simulink model "robust_drift_REALTIME"  (R2020b)
settings: Solver=VariableStepAuto  StartTime=0.0  StopTime=10.0  RelTol=1e-3
values from neighbouring files (symbols this model uses):
  drv =     [balrob_params.mat]
  gbox =     [balrob_params.mat]    (also in sfun_balrob_long_dyn.m = block.DialogPrm(4).Data)
  sens =     [balrob_params.mat]
  Ts = 0.01    [balrob_params.mat]
  wheel =     [balrob_params.mat]    (also in sfun_balrob_long_dyn.m = block.DialogPrm(5).Data)
undefined symbols (not defined in the file or in its folder): C_gain, denHw, denLPFz, DiscIntNeverNeededParam, Ki, N_u, N_x, numHw, numLPFz, T
settings Model: Creator=39345  LastModifiedBy=39345

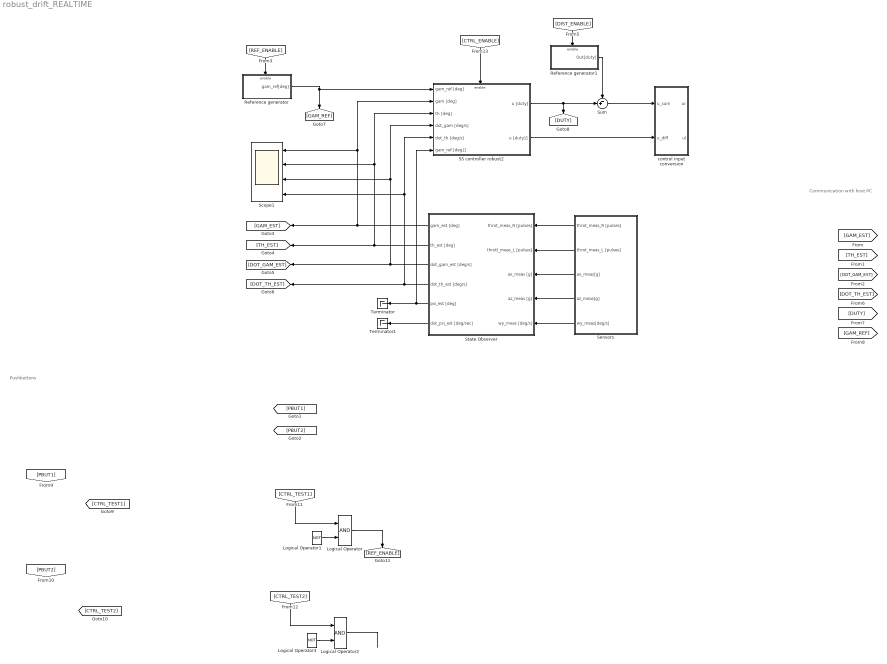
== system robust_drift_REALTIME ==
  note: Communication with host PC
  note: Pushbuttons
  Logical Operator : Logic  AllPortsSameDT=off  OutDataTypeStr=boolean
  Logical Operator1 : Logic  Operator=NOT  Inputs=1  AllPortsSameDT=off  OutDataTypeStr=boolean
  Logical Operator2 : Logic  AllPortsSameDT=off  OutDataTypeStr=boolean
  Logical Operator3 : Logic  Operator=NOT  Inputs=1  AllPortsSameDT=off  OutDataTypeStr=boolean
  Reference generator : Subsystem
  Reference generator1 : Subsystem
  SS controller robust2 : Subsystem
  Scope1 : Scope  NumInputPorts=4
  Sensors : Subsystem
  State Observer : Subsystem
  Sum : Sum  Inputs=-+|
  Terminator : Terminator
  Terminator1 : Terminator
  control input conversion : Subsystem
  wires:
  Logical Operator/1 -> [REF_ENABLE]
  [CTRL_TEST1] -> Logical Operator/1
  Logical Operator2/1 -> ?
  Logical Operator1/1 -> Logical Operator/2
  [CTRL_TEST2] -> Logical Operator2/1
  Logical Operator3/1 -> Logical Operator2/2
  [CTRL_ENABLE] -> SS controller robust2/Enable
  State Observer/5(psi_est [deg]) -> SS controller robust2/6(gam_ref [deg]1), Terminator/1
  [REF_ENABLE] -> Reference generator/Enable
  State Observer/1(gam_est [deg]) -> SS controller robust2/2(gam [deg]), Scope1/1, [GAM_EST]
  Sensors/3(ax_meas[g]) -> State Observer/3("ax_meas [g] ")
  State Observer/2(th_est [deg]) -> SS controller robust2/3(th [deg]), Scope1/2, [TH_EST]
  Sensors/4(az_meas[g]) -> State Observer/4("az_meas [g] ")
  Reference generator/1(gam_ref[deg]) -> SS controller robust2/1(gam_ref [deg]), [GAM_REF]
  Sum/1 -> control input conversion/1(u_sum)
  Sensors/2(throt_meas_L [pulses]) -> State Observer/2(throtl_meas_L [pulses])
  State Observer/4(dot_th_est [deg/s]) -> SS controller robust2/5(dot_th [deg/s]), Scope1/4, [DOT_TH_EST]
  Reference generator1/1(Out[duty]) -> Sum/1
  State Observer/6(dot_psi_est [deg/sec]) -> Terminator1/1
  Sensors/1(throt_meas_R [pulses]) -> State Observer/1("throt_meas_R [pulses] ")
  State Observer/3(dot_gam_est [deg/s]) -> SS controller robust2/4(dot_gam [deg/s]), Scope1/3, [DOT_GAM_EST]
  Sensors/5(wy_meas[deg/s]) -> State Observer/5(wy_meas [deg/s])
  [DIST_ENABLE] -> Reference generator1/Enable
  SS controller robust2/1(u [duty]) -> Sum/2, [DUTY]
  SS controller robust2/2(u [duty]1) -> control input conversion/2(u_diff)

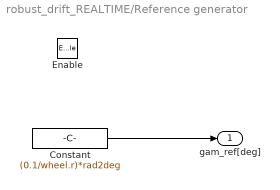
== system robust_drift_REALTIME/Reference generator ==
  Enable : EnablePort  StatesWhenEnabling=reset
  Constant : Constant  Value=(0.1/wheel.r)*rad2deg
  gam_ref[deg] : Outport
  wires:
  Constant/1 -> gam_ref[deg]/1

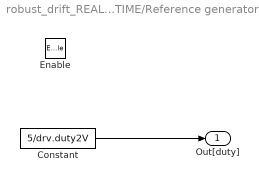
== system robust_drift_REALTIME/Reference generator1 ==
  Enable : EnablePort  StatesWhenEnabling=reset
  Constant : Constant  Value=5/drv.duty2V
  Out[duty] : Outport
  wires:
  Constant/1 -> Out[duty]/1

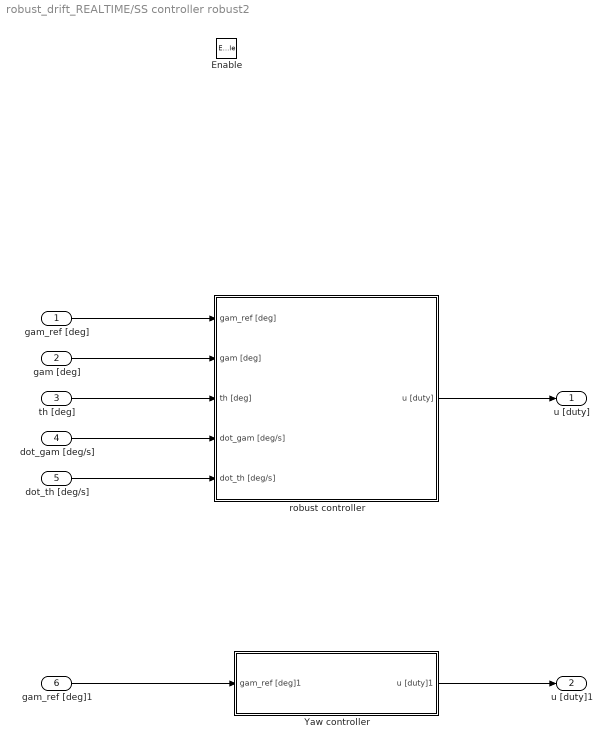
== system robust_drift_REALTIME/SS controller robust2 ==
  gam_ref [deg] : Inport
  gam [deg] : Inport  Port=2
  th [deg] : Inport  Port=3
  dot_gam [deg/s] : Inport  Port=4
  dot_th [deg/s] : Inport  Port=5
  gam_ref [deg]1 : Inport  Port=6
  Enable : EnablePort
  Yaw controller : Subsystem
  robust controller : Subsystem
  u [duty] : Outport
  u [duty]1 : Outport  Port=2
  wires:
  gam_ref [deg]1/1 -> Yaw controller/1(gam_ref [deg]1)
  Yaw controller/1(u [duty]1) -> u [duty]1/1
  gam_ref [deg]/1 -> robust controller/1(gam_ref [deg])
  robust controller/1(u [duty]) -> u [duty]/1
  gam [deg]/1 -> robust controller/2(gam [deg])
  th [deg]/1 -> robust controller/3(th [deg])
  dot_gam [deg/s]/1 -> robust controller/4(dot_gam [deg/s])
  dot_th [deg/s]/1 -> robust controller/5(dot_th [deg/s])

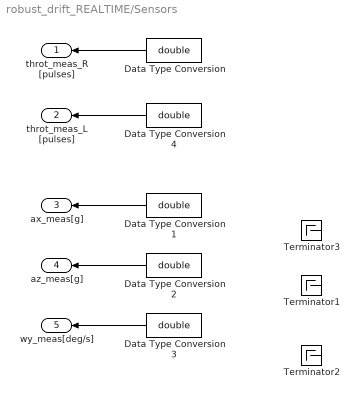
== system robust_drift_REALTIME/Sensors ==
  Data Type Conversion{,1..4} (5 alike) : DataTypeConversion  OutDataTypeStr=double
  Terminator1 : Terminator
  Terminator2 : Terminator
  Terminator3 : Terminator
  throt_meas_R [pulses] : Outport
  throt_meas_L [pulses] : Outport  Port=2
  ax_meas[g] : Outport  Port=3
  az_meas[g] : Outport  Port=4
  wy_meas[deg/s] : Outport  Port=5
  wires:
  Data Type Conversion/1 -> throt_meas_R [pulses]/1
  Data Type Conversion1/1 -> ax_meas[g]/1
  Data Type Conversion2/1 -> az_meas[g]/1
  Data Type Conversion3/1 -> wy_meas[deg/s]/1
  Data Type Conversion4/1 -> throt_meas_L [pulses]/1

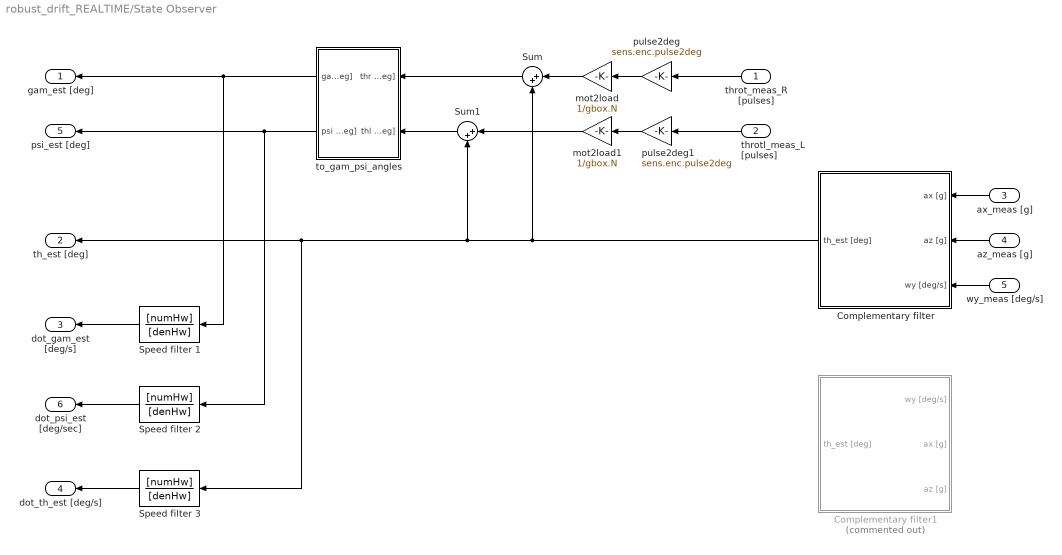
== system robust_drift_REALTIME/State Observer ==
  "throt_meas_R [pulses] " : Inport
  throtl_meas_L [pulses] : Inport  Port=2
  "ax_meas [g] " : Inport  Port=3
  "az_meas [g] " : Inport  Port=4
  wy_meas [deg/s] : Inport  Port=5
  Complementary filter : Subsystem
  Complementary filter1 : Subsystem  Commented=on
  Speed filter 1 : DiscreteTransferFcn  Numerator=[numHw]  Denominator=[denHw]  SampleTime=Ts
  Speed filter 2 : DiscreteTransferFcn  Numerator=[numHw]  Denominator=[denHw]  SampleTime=Ts
  Speed filter 3 : DiscreteTransferFcn  Numerator=[numHw]  Denominator=[denHw]  SampleTime=Ts
  Sum : Sum  Inputs=|++
  Sum1 : Sum  Inputs=|++
  mot2load : Gain  Gain=1/gbox.N
  mot2load1 : Gain  Gain=1/gbox.N
  pulse2deg : Gain  Gain=sens.enc.pulse2deg
  pulse2deg1 : Gain  Gain=sens.enc.pulse2deg
  to_gam_psi_angles : Subsystem
  gam_est [deg] : Outport
  th_est [deg] : Outport  Port=2
  dot_gam_est [deg/s] : Outport  Port=3
  dot_th_est [deg/s] : Outport  Port=4
  psi_est [deg] : Outport  Port=5
  dot_psi_est [deg/sec] : Outport  Port=6
  wires:
  pulse2deg/1 -> mot2load/1
  "throt_meas_R [pulses] "/1 -> pulse2deg/1
  mot2load/1 -> Sum/1
  Complementary filter/1("th_est [deg] ") -> Sum/2, th_est [deg]/1, Speed filter 3/1, Sum1/2
  Speed filter 1/1 -> dot_gam_est [deg/s]/1
  Speed filter 3/1 -> dot_th_est [deg/s]/1
  "ax_meas [g] "/1 -> Complementary filter/1("ax [g] ")
  "az_meas [g] "/1 -> Complementary filter/2("az [g] ")
  wy_meas [deg/s]/1 -> Complementary filter/3(wy [deg/s])
  throtl_meas_L [pulses]/1 -> pulse2deg1/1
  pulse2deg1/1 -> mot2load1/1
  mot2load1/1 -> Sum1/1
  Sum1/1 -> to_gam_psi_angles/2(thl [deg])
  Sum/1 -> to_gam_psi_angles/1(thr [deg])
  to_gam_psi_angles/1(gam [deg]) -> Speed filter 1/1, gam_est [deg]/1
  to_gam_psi_angles/2(psi [deg]) -> Speed filter 2/1, psi_est [deg]/1
  Speed filter 2/1 -> dot_psi_est [deg/sec]/1

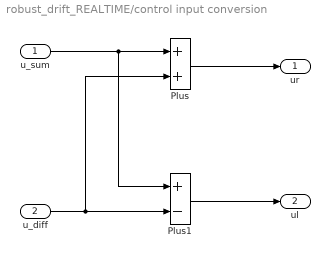
== system robust_drift_REALTIME/control input conversion ==
  u_sum : Inport
  u_diff : Inport  Port=2
  Plus : Sum
  Plus1 : Sum  Inputs=+-
  ur : Outport
  ul : Outport  Port=2
  wires:
  u_sum/1 -> Plus1/1, Plus/1
  u_diff/1 -> Plus1/2, Plus/2
  Plus/1 -> ur/1
  Plus1/1 -> ul/1

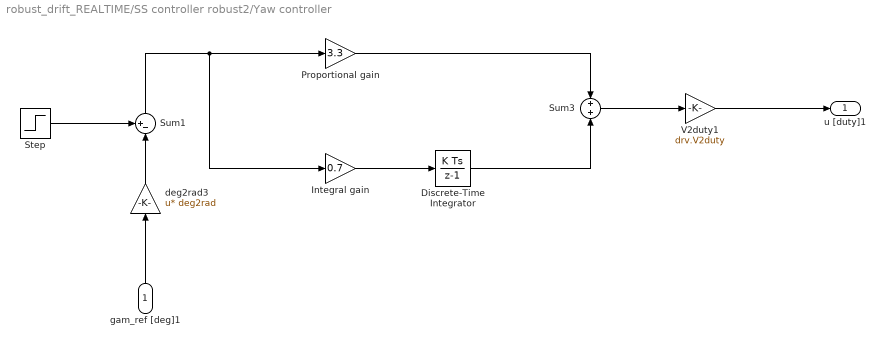
== system robust_drift_REALTIME/SS controller robust2/Yaw controller ==
  gam_ref [deg]1 : Inport
  Discrete-Time Integrator : DiscreteIntegrator  SampleTime=-1  ICPrevOutput=DiscIntNeverNeededParam  ICPrevScaledInput=DiscIntNeverNeededParam
  Integral gain : Gain  Gain=0.7
  Proportional gain : Gain  Gain=3.3
  Step : Step  Time=0  After=0  SampleTime=0
  Sum1 : Sum  Inputs=+-|
  Sum3 : Sum  Inputs=+|+
  V2duty1 : Gain  Gain=drv.V2duty
  deg2rad3 : Gain  Gain=deg2rad  Multiplication=Matrix(u*K)
  u [duty]1 : Outport
  wires:
  gam_ref [deg]1/1 -> deg2rad3/1
  Sum1/1 -> Integral gain/1, Proportional gain/1
  Step/1 -> Sum1/1
  Integral gain/1 -> Discrete-Time Integrator/1
  deg2rad3/1 -> Sum1/2
  V2duty1/1 -> u [duty]1/1
  Proportional gain/1 -> Sum3/1
  Discrete-Time Integrator/1 -> Sum3/2
  Sum3/1 -> V2duty1/1

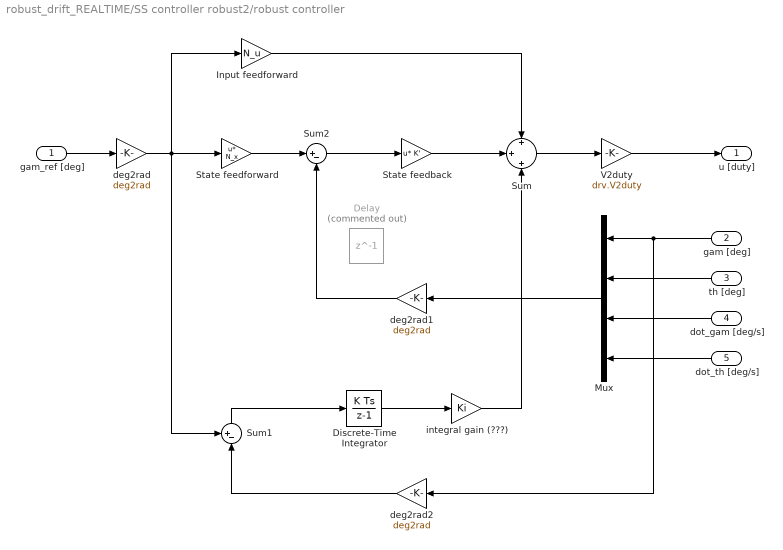
== system robust_drift_REALTIME/SS controller robust2/robust controller ==
  gam_ref [deg] : Inport
  gam [deg] : Inport  Port=2
  th [deg] : Inport  Port=3
  dot_gam [deg/s] : Inport  Port=4
  dot_th [deg/s] : Inport  Port=5
  Delay : Delay  Commented=on  DelayLength=1  InitialCondition=0
  Discrete-Time Integrator : DiscreteIntegrator  SampleTime=0.01  ICPrevOutput=DiscIntNeverNeededParam  ICPrevScaledInput=DiscIntNeverNeededParam
  Input feedforward : Gain  Gain=N_u
  Mux : Mux
  State feedback : Gain  Gain=K'  Multiplication=Matrix(u*K)
  "State feedforward\t" : Gain  Gain=N_x  Multiplication=Matrix(u*K)
  Sum : Sum  Inputs=+|+|+
  Sum1 : Sum  Inputs=+-|
  Sum2 : Sum  Inputs=|+-
  V2duty : Gain  Gain=drv.V2duty
  deg2rad : Gain  Gain=deg2rad
  deg2rad1 : Gain  Gain=deg2rad
  deg2rad2 : Gain  Gain=deg2rad
  integral gain (???) : Gain  Gain=Ki
  u [duty] : Outport
  wires:
  integral gain (???)/1 -> Sum/3
  deg2rad2/1 -> Sum1/2
  Sum1/1 -> Discrete-Time Integrator/1
  deg2rad/1 -> Sum1/1, "State feedforward\t"/1, Input feedforward/1
  Input feedforward/1 -> Sum/1
  Discrete-Time Integrator/1 -> integral gain (???)/1
  gam_ref [deg]/1 -> deg2rad/1
  Sum2/1 -> State feedback/1
  Mux/1 -> deg2rad1/1
  gam [deg]/1 -> deg2rad2/1, Mux/1
  dot_gam [deg/s]/1 -> Mux/3
  dot_th [deg/s]/1 -> Mux/4
  "State feedforward\t"/1 -> Sum2/1
  Sum/1 -> V2duty/1
  State feedback/1 -> Sum/2
  th [deg]/1 -> Mux/2
  deg2rad1/1 -> Sum2/2
  V2duty/1 -> u [duty]/1

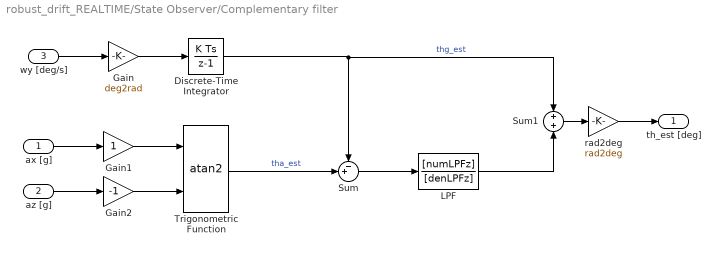
== system robust_drift_REALTIME/State Observer/Complementary filter ==
  "ax [g] " : Inport
  "az [g] " : Inport  Port=2
  wy [deg/s] : Inport  Port=3
  Discrete-Time Integrator : DiscreteIntegrator  gainval=1  SampleTime=Ts  ICPrevOutput=DiscIntNeverNeededParam  ICPrevScaledInput=DiscIntNeverNeededParam
  Gain : Gain  Gain=deg2rad
  Gain1 : Gain
  Gain2 : Gain  Gain=-1
  LPF : DiscreteTransferFcn  Numerator=[numLPFz]  Denominator=[denLPFz]  SampleTime=Ts
  Sum : Sum  Inputs=-+|
  Sum1 : Sum
  Trigonometric Function : Trigonometry  Operator=atan2
  rad2deg : Gain  Gain=rad2deg
  "th_est [deg] " : Outport
  wires:
  "az [g] "/1 -> Gain2/1
  "ax [g] "/1 -> Gain1/1
  wy [deg/s]/1 -> Gain/1
  Gain/1 -> Discrete-Time Integrator/1
  Gain2/1 -> Trigonometric Function/2
  Gain1/1 -> Trigonometric Function/1
  Trigonometric Function/1 -> Sum/2  "tha_est"
  Discrete-Time Integrator/1 -> Sum1/1, Sum/1  "thg_est"
  rad2deg/1 -> "th_est [deg] "/1
  Sum1/1 -> rad2deg/1
  Sum/1 -> LPF/1
  LPF/1 -> Sum1/2

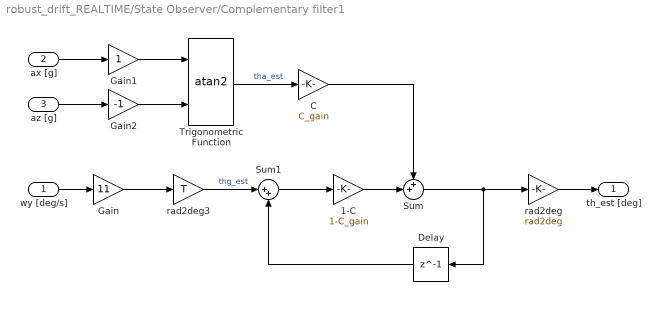
== system robust_drift_REALTIME/State Observer/Complementary filter1 ==
  wy [deg/s] : Inport
  "ax [g] " : Inport  Port=2
  "az [g] " : Inport  Port=3
  1-C : Gain  Gain=1-C_gain
  C : Gain  Gain=C_gain
  Delay : Delay  DelayLength=1
  Gain : Gain  Gain=11
  Gain1 : Gain
  Gain2 : Gain  Gain=-1
  Sum : Sum  Inputs=++|
  Sum1 : Sum  Inputs=|++
  Trigonometric Function : Trigonometry  Operator=atan2
  rad2deg : Gain  Gain=rad2deg
  rad2deg3 : Gain  Gain=T
  "th_est [deg] " : Outport
  wires:
  "az [g] "/1 -> Gain2/1
  "ax [g] "/1 -> Gain1/1
  wy [deg/s]/1 -> Gain/1
  Gain/1 -> rad2deg3/1
  Gain2/1 -> Trigonometric Function/2
  Gain1/1 -> Trigonometric Function/1
  rad2deg/1 -> "th_est [deg] "/1
  Trigonometric Function/1 -> C/1  "tha_est"
  C/1 -> Sum/1
  1-C/1 -> Sum/2
  Sum/1 -> Delay/1, rad2deg/1
  Delay/1 -> Sum1/2
  rad2deg3/1 -> Sum1/1  "thg_est"
  Sum1/1 -> 1-C/1

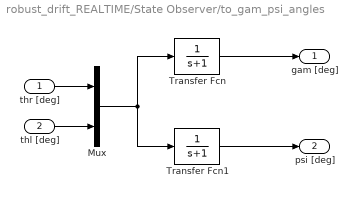
== system robust_drift_REALTIME/State Observer/to_gam_psi_angles ==
  thr [deg] : Inport
  thl [deg] : Inport  Port=2
  Mux : Mux  Inputs=2
  Transfer Fcn : TransferFcn  Denominator=[1 1]
  Transfer Fcn1 : TransferFcn  Denominator=[1 1]
  gam [deg] : Outport
  psi [deg] : Outport  Port=2
  wires:
  thr [deg]/1 -> Mux/1
  thl [deg]/1 -> Mux/2
  Mux/1 -> Transfer Fcn1/1, Transfer Fcn/1
  Transfer Fcn/1 -> gam [deg]/1
  Transfer Fcn1/1 -> psi [deg]/1
